simulink model "Electrolyzer"  (R2025b)
settings: Solver=VariableStepAuto  StartTime=0.0  StopTime=10.0  RelTol=1e-3
undefined symbols (not defined in the file): alpha, beta, E0, k_deg, R0_init, T0

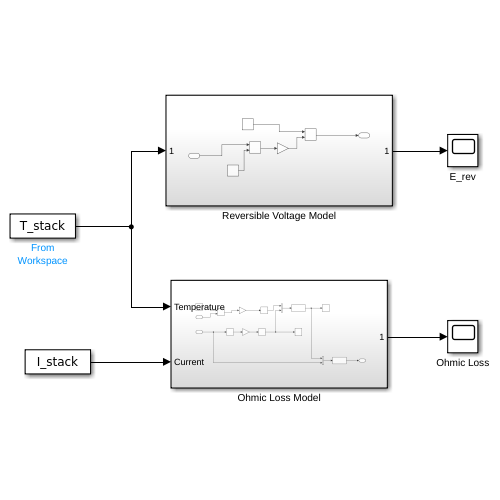
[thumbnail: Simulink's stored preview of the top-level diagram]
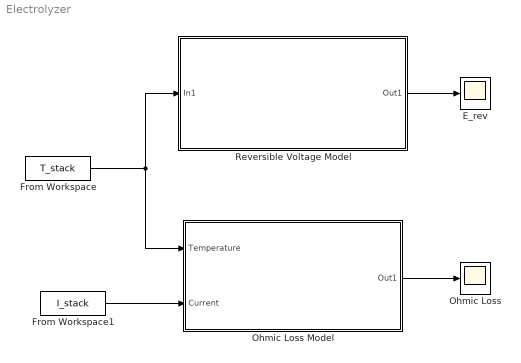
== system Electrolyzer ==
  E_rev : Scope
  From Workspace : FromWorkspace  VariableName=T_stack
  From Workspace1 : FromWorkspace  VariableName=I_stack
  Ohmic Loss : Scope
      settings: DataLoggingVariableName=ScopeData3
  Ohmic Loss Model : Subsystem
  Reversible Voltage Model : Subsystem
  wires:
  From Workspace/1 -> Reversible Voltage Model/1(In1), Ohmic Loss Model/1(Temperature)
  Reversible Voltage Model/1(Out1) -> E_rev/1
  Ohmic Loss Model/1(Out1) -> Ohmic Loss/1
  From Workspace1/1 -> Ohmic Loss Model/2(Current)

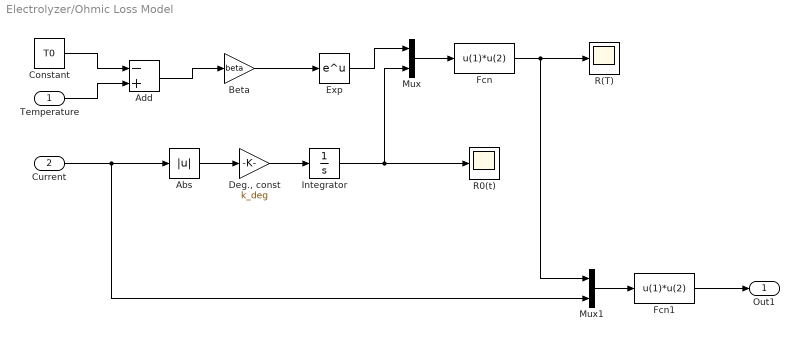
== system Electrolyzer/Ohmic Loss Model ==
  Temperature : Inport
  Current : Inport  Port=2
  Abs : Abs  SaturateOnIntegerOverflow=off
  Add : Sum  Inputs=-+
  Beta : Gain  Gain=beta
  Constant : Constant  Value=T0
  "Deg., const" : Gain  Gain=k_deg
  Exp : Math
  Fcn : Fcn  Expr=u(1)*u(2)
  Fcn1 : Fcn  Expr=u(1)*u(2)
  Integrator : Integrator  InitialCondition=R0_init
  Mux : Mux  Inputs=2
  Mux1 : Mux  Inputs=2
  R(T) : Scope
      settings: DataLoggingVariableName=ScopeData2
  R0(t) : Scope
  Out1 : Outport
  wires:
  Abs/1 -> "Deg., const"/1
  Integrator/1 -> Mux/2, R0(t)/1
  "Deg., const"/1 -> Integrator/1
  Current/1 -> Mux1/2, Abs/1
  Temperature/1 -> Add/2
  Constant/1 -> Add/1
  Add/1 -> Beta/1
  Beta/1 -> Exp/1
  Exp/1 -> Mux/1
  Mux/1 -> Fcn/1
  Fcn/1 -> Mux1/1, R(T)/1
  Mux1/1 -> Fcn1/1
  Fcn1/1 -> Out1/1

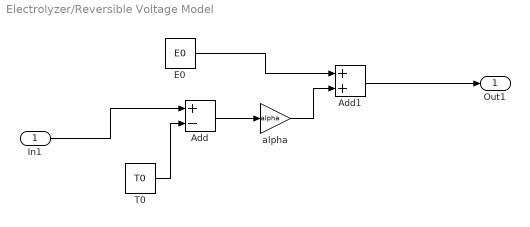
== system Electrolyzer/Reversible Voltage Model ==
  In1 : Inport
  Add : Sum  Inputs=+-
  Add1 : Sum
  E0 : Constant  Value=E0
  T0 : Constant  Value=T0
  alpha : Gain  Gain=alpha
  Out1 : Outport
  wires:
  Add/1 -> alpha/1
  E0/1 -> Add1/1
  alpha/1 -> Add1/2
  In1/1 -> Add/1
  T0/1 -> Add/2
  Add1/1 -> Out1/1
